simulink model "controllo_giunti_2"  (R2020b)
settings: Solver=FixedStepAuto  StartTime=0.0  StopTime=1  FixedStep=0.001  RelTol=1e-3
libraries: robotcorelib x1
(part 2 of 2)

== matlab function controllo_giunti_2/Subsystem/dq3_dq4 ==
  data: Q input; dQ input; dq3 output; parametri input; dq4 output
function [dq3,dq4] = dq3_dq4(Q,dQ,parametri)
xc1=Q(1);
xc5=Q(2);
q2=Q(3);
dxc1=dQ(1);
dxc5=dQ(2);
dq2=dQ(3);
l=parametri(1);

dq3 =...
(2*dxc5*((2*l + (4*sin(q2)*l^3 - 4*sin(2*q2)*l^2*xc1 - 4*cos(2*q2)*l^2*xc5 - 4*sin(q2)*l*xc1^2 + 8*cos(q2)*l*xc1*xc5 - 12*sin(q2)*l*xc5^2 + 4*xc1^2*xc5 + 4*xc5^3)/(2*(3*l^4 + 4*cos(q2)*l^3*xc1 - 4*sin(q2)*l^3*xc5 - 2*cos(2*q2)*l^2*xc1^2 + 4*sin(2*q2)*l^2*xc1*xc5 + 2*cos(2*q2)*l^2*xc5^2 - 4*cos(q2)*l*xc1^3 + 4*sin(q2)*l*xc1^2*xc5 - 4*cos(q2)*l*xc1*xc5^2 + 4*sin(q2)*l*xc5^3 - xc1^4 - 2*xc1^2*xc5^2 - xc5^4)^(1/2)))/(l^2 - 2*l*xc1 + xc1^2 + xc5^2 - 2*l^2*cos(q2) + 2*l*xc1*cos(q2) - 2*l*xc5*sin(q2)) + ((2*xc5 - 2*l*sin(q2))*(2*l^2*sin(q2) + (3*l^4 + 4*cos(q2)*l^3*xc1 - 4*sin(q2)*l^3*xc5 - 2*cos(2*q2)*l^2*xc1^2 + 4*sin(2*q2)*l^2*xc1*xc5 + 2*cos(2*q2)*l^2*xc5^2 - 4*cos(q2)*l*xc1^3 + 4*sin(q2)*l*xc1^2*xc5 - 4*cos(q2)*l*xc1*xc5^2 + 4*sin(q2)*l*xc5^3 - xc1^4 - 2*xc1^2*xc5^2 - xc5^4)^(1/2) - 2*l*xc5))/(l^2 - 2*l*xc1 + xc1^2 + xc5^2 - 2*l^2*cos(q2) + 2*l*xc1*cos(q2) - 2*l*xc5*sin(q2))^2))/((2*l^2*sin(q2) + (3*l^4 + 4*cos(q2)*l^3*xc1 - 4*sin(q2)*l^3*xc5 - 2*cos(2*q2)*l^2*xc1^2 + 4*sin(2*q2)*l^2*xc1*xc5 + 2*cos(2*q2)*l^2*xc5^2 - 4*cos(q2)*l*xc1^3 + 4*sin(q2)*l*xc1^2*xc5 - 4*cos(q2)*l*xc1*xc5^2 + 4*sin(q2)*l*xc5^3 - xc1^4 - 2*xc1^2*xc5^2 - xc5^4)^(1/2) - 2*l*xc5)^2/(l^2 - 2*l*xc1 + xc1^2 + xc5^2 - 2*l^2*cos(q2) + 2*l*xc1*cos(q2) - 2*l*xc5*sin(q2))^2 + 1) - dq2*((2*(((- 4*sin(q2)*l^3*xc1 - 4*cos(q2)*l^3*xc5 + 4*sin(2*q2)*l^2*xc1^2 + 8*cos(2*q2)*l^2*xc1*xc5 - 4*sin(2*q2)*l^2*xc5^2 + 4*sin(q2)*l*xc1^3 + 4*cos(q2)*l*xc1^2*xc5 + 4*sin(q2)*l*xc1*xc5^2 + 4*cos(q2)*l*xc5^3)/(2*(3*l^4 + 4*cos(q2)*l^3*xc1 - 4*sin(q2)*l^3*xc5 - 2*cos(2*q2)*l^2*xc1^2 + 4*sin(2*q2)*l^2*xc1*xc5 + 2*cos(2*q2)*l^2*xc5^2 - 4*cos(q2)*l*xc1^3 + 4*sin(q2)*l*xc1^2*xc5 - 4*cos(q2)*l*xc1*xc5^2 + 4*sin(q2)*l*xc5^3 - xc1^4 - 2*xc1^2*xc5^2 - xc5^4)^(1/2)) + 2*l^2*cos(q2))/(l^2 - 2*l*xc1 + xc1^2 + xc5^2 - 2*l^2*cos(q2) + 2*l*xc1*cos(q2) - 2*l*xc5*sin(q2)) + ((2*l*xc5*cos(q2) - 2*l^2*sin(q2) + 2*l*xc1*sin(q2))*(2*l^2*sin(q2) + (3*l^4 + 4*cos(q2)*l^3*xc1 - 4*sin(q2)*l^3*xc5 - 2*cos(2*q2)*l^2*xc1^2 + 4*sin(2*q2)*l^2*xc1*xc5 + 2*cos(2*q2)*l^2*xc5^2 - 4*cos(q2)*l*xc1^3 + 4*sin(q2)*l*xc1^2*xc5 - 4*cos(q2)*l*xc1*xc5^2 + 4*sin(q2)*l*xc5^3 - xc1^4 - 2*xc1^2*xc5^2 - xc5^4)^(1/2) - 2*l*xc5))/(l^2 - 2*l*xc1 + xc1^2 + xc5^2 - 2*l^2*cos(q2) + 2*l*xc1*cos(q2) - 2*l*xc5*sin(q2))^2))/((2*l^2*sin(q2) + (3*l^4 + 4*cos(q2)*l^3*xc1 - 4*sin(q2)*l^3*xc5 - 2*cos(2*q2)*l^2*xc1^2 + 4*sin(2*q2)*l^2*xc1*xc5 + 2*cos(2*q2)*l^2*xc5^2 - 4*cos(q2)*l*xc1^3 + 4*sin(q2)*l*xc1^2*xc5 - 4*cos(q2)*l*xc1*xc5^2 + 4*sin(q2)*l*xc5^3 - xc1^4 - 2*xc1^2*xc5^2 - xc5^4)^(1/2) - 2*l*xc5)^2/(l^2 - 2*l*xc1 + xc1^2 + xc5^2 - 2*l^2*cos(q2) + 2*l*xc1*cos(q2) - 2*l*xc5*sin(q2))^2 + 1) + 1) + (2*dxc1*(((2*xc1 - 2*l + 2*l*cos(q2))*(2*l^2*sin(q2) + (3*l^4 + 4*cos(q2)*l^3*xc1 - 4*sin(q2)*l^3*xc5 - 2*cos(2*q2)*l^2*xc1^2 + 4*sin(2*q2)*l^2*xc1*xc5 + 2*cos(2*q2)*l^2*xc5^2 - 4*cos(q2)*l*xc1^3 + 4*sin(q2)*l*xc1^2*xc5 - 4*cos(q2)*l*xc1*xc5^2 + 4*sin(q2)*l*xc5^3 - xc1^4 - 2*xc1^2*xc5^2 - xc5^4)^(1/2) - 2*l*xc5))/(l^2 - 2*l*xc1 + xc1^2 + xc5^2 - 2*l^2*cos(q2) + 2*l*xc1*cos(q2) - 2*l*xc5*sin(q2))^2 + (- 4*cos(q2)*l^3 + 4*cos(2*q2)*l^2*xc1 - 4*sin(2*q2)*l^2*xc5 + 12*cos(q2)*l*xc1^2 - 8*sin(q2)*l*xc1*xc5 + 4*cos(q2)*l*xc5^2 + 4*xc1^3 + 4*xc1*xc5^2)/(2*(l^2 - 2*l*xc1 + xc1^2 + xc5^2 - 2*l^2*cos(q2) + 2*l*xc1*cos(q2) - 2*l*xc5*sin(q2))*(3*l^4 + 4*cos(q2)*l^3*xc1 - 4*sin(q2)*l^3*xc5 - 2*cos(2*q2)*l^2*xc1^2 + 4*sin(2*q2)*l^2*xc1*xc5 + 2*cos(2*q2)*l^2*xc5^2 - 4*cos(q2)*l*xc1^3 + 4*sin(q2)*l*xc1^2*xc5 - 4*cos(q2)*l*xc1*xc5^2 + 4*sin(q2)*l*xc5^3 - xc1^4 - 2*xc1^2*xc5^2 - xc5^4)^(1/2))))/((2*l^2*sin(q2) + (3*l^4 + 4*cos(q2)*l^3*xc1 - 4*sin(q2)*l^3*xc5 - 2*cos(2*q2)*l^2*xc1^2 + 4*sin(2*q2)*l^2*xc1*xc5 + 2*cos(2*q2)*l^2*xc5^2 - 4*cos(q2)*l*xc1^3 + 4*sin(q2)*l*xc1^2*xc5 - 4*cos(q2)*l*xc1*xc5^2 + 4*sin(q2)*l*xc5^3 - xc1^4 - 2*xc1^2*xc5^2 - xc5^4)^(1/2) - 2*l*xc5)^2/(l^2 - 2*l*xc1 + xc1^2 + xc5^2 - 2*l^2*cos(q2) + 2*l*xc1*cos(q2) - 2*l*xc5*sin(q2))^2 + 1);

dq4 =...
 - dxc1*((2*(((2*xc1 - 2*l + 2*l*cos(q2))*((3*l^4 + 4*cos(q2)*l^3*xc1 - 4*sin(q2)*l^3*xc5 - 2*cos(2*q2)*l^2*xc1^2 + 4*sin(2*q2)*l^2*xc1*xc5 + 2*cos(2*q2)*l^2*xc5^2 - 4*cos(q2)*l*xc1^3 + 4*sin(q2)*l*xc1^2*xc5 - 4*cos(q2)*l*xc1*xc5^2 + 4*sin(q2)*l*xc5^3 - xc1^4 - 2*xc1^2*xc5^2 - xc5^4)^(1/2) - 2*l^2*sin(q2) + 2*l*xc5))/(l^2 - 2*l*xc1 + xc1^2 + xc5^2 - 2*l^2*cos(q2) + 2*l*xc1*cos(q2) - 2*l*xc5*sin(q2))^2 + (2*(xc1 + l*cos(q2))*(- l^2 + 2*cos(q2)*l*xc1 - 2*sin(q2)*l*xc5 + xc1^2 + xc5^2))/((l^2 - 2*l*xc1 + xc1^2 + xc5^2 - 2*l^2*cos(q2) + 2*l*xc1*cos(q2) - 2*l*xc5*sin(q2))*(3*l^4 + 4*cos(q2)*l^3*xc1 - 4*sin(q2)*l^3*xc5 - 2*cos(2*q2)*l^2*xc1^2 + 4*sin(2*q2)*l^2*xc1*xc5 + 2*cos(2*q2)*l^2*xc5^2 - 4*cos(q2)*l*xc1^3 + 4*sin(q2)*l*xc1^2*xc5 - 4*cos(q2)*l*xc1*xc5^2 + 4*sin(q2)*l*xc5^3 - xc1^4 - 2*xc1^2*xc5^2 - xc5^4)^(1/2))))/(((3*l^4 + 4*cos(q2)*l^3*xc1 - 4*sin(q2)*l^3*xc5 - 2*cos(2*q2)*l^2*xc1^2 + 4*sin(2*q2)*l^2*xc1*xc5 + 2*cos(2*q2)*l^2*xc5^2 - 4*cos(q2)*l*xc1^3 + 4*sin(q2)*l*xc1^2*xc5 - 4*cos(q2)*l*xc1*xc5^2 + 4*sin(q2)*l*xc5^3 - xc1^4 - 2*xc1^2*xc5^2 - xc5^4)^(1/2) - 2*l^2*sin(q2) + 2*l*xc5)^2/(l^2 - 2*l*xc1 + xc1^2 + xc5^2 - 2*l^2*cos(q2) + 2*l*xc1*cos(q2) - 2*l*xc5*sin(q2))^2 + 1) + (2*(((2*xc1 - 2*l + 2*l*cos(q2))*(2*l^2*sin(q2) + (3*l^4 + 4*cos(q2)*l^3*xc1 - 4*sin(q2)*l^3*xc5 - 2*cos(2*q2)*l^2*xc1^2 + 4*sin(2*q2)*l^2*xc1*xc5 + 2*cos(2*q2)*l^2*xc5^2 - 4*cos(q2)*l*xc1^3 + 4*sin(q2)*l*xc1^2*xc5 - 4*cos(q2)*l*xc1*xc5^2 + 4*sin(q2)*l*xc5^3 - xc1^4 - 2*xc1^2*xc5^2 - xc5^4)^(1/2) - 2*l*xc5))/(l^2 - 2*l*xc1 + xc1^2 + xc5^2 - 2*l^2*cos(q2) + 2*l*xc1*cos(q2) - 2*l*xc5*sin(q2))^2 + (2*(xc1 + l*cos(q2))*(- l^2 + 2*cos(q2)*l*xc1 - 2*sin(q2)*l*xc5 + xc1^2 + xc5^2))/((l^2 - 2*l*xc1 + xc1^2 + xc5^2 - 2*l^2*cos(q2) + 2*l*xc1*cos(q2) - 2*l*xc5*sin(q2))*(3*l^4 + 4*cos(q2)*l^3*xc1 - 4*sin(q2)*l^3*xc5 - 2*cos(2*q2)*l^2*xc1^2 + 4*sin(2*q2)*l^2*xc1*xc5 + 2*cos(2*q2)*l^2*xc5^2 - 4*cos(q2)*l*xc1^3 + 4*sin(q2)*l*xc1^2*xc5 - 4*cos(q2)*l*xc1*xc5^2 + 4*sin(q2)*l*xc5^3 - xc1^4 - 2*xc1^2*xc5^2 - xc5^4)^(1/2))))/((2*l^2*sin(q2) + (3*l^4 + 4*cos(q2)*l^3*xc1 - 4*sin(q2)*l^3*xc5 - 2*cos(2*q2)*l^2*xc1^2 + 4*sin(2*q2)*l^2*xc1*xc5 + 2*cos(2*q2)*l^2*xc5^2 - 4*cos(q2)*l*xc1^3 + 4*sin(q2)*l*xc1^2*xc5 - 4*cos(q2)*l*xc1*xc5^2 + 4*sin(q2)*l*xc5^3 - xc1^4 - 2*xc1^2*xc5^2 - xc5^4)^(1/2) - 2*l*xc5)^2/(l^2 - 2*l*xc1 + xc1^2 + xc5^2 - 2*l^2*cos(q2) + 2*l*xc1*cos(q2) - 2*l*xc5*sin(q2))^2 + 1)) - dxc5*((2*((2*l + (2*sin(q2)*l^3 - 2*sin(2*q2)*l^2*xc1 - 2*cos(2*q2)*l^2*xc5 - 2*sin(q2)*l*xc1^2 + 4*cos(q2)*l*xc1*xc5 - 6*sin(q2)*l*xc5^2 + 2*xc1^2*xc5 + 2*xc5^3)/(3*l^4 + 4*cos(q2)*l^3*xc1 - 4*sin(q2)*l^3*xc5 - 2*cos(2*q2)*l^2*xc1^2 + 4*sin(2*q2)*l^2*xc1*xc5 + 2*cos(2*q2)*l^2*xc5^2 - 4*cos(q2)*l*xc1^3 + 4*sin(q2)*l*xc1^2*xc5 - 4*cos(q2)*l*xc1*xc5^2 + 4*sin(q2)*l*xc5^3 - xc1^4 - 2*xc1^2*xc5^2 - xc5^4)^(1/2))/(l^2 - 2*l*xc1 + xc1^2 + xc5^2 - 2*l^2*cos(q2) + 2*l*xc1*cos(q2) - 2*l*xc5*sin(q2)) + ((2*xc5 - 2*l*sin(q2))*(2*l^2*sin(q2) + (3*l^4 + 4*cos(q2)*l^3*xc1 - 4*sin(q2)*l^3*xc5 - 2*cos(2*q2)*l^2*xc1^2 + 4*sin(2*q2)*l^2*xc1*xc5 + 2*cos(2*q2)*l^2*xc5^2 - 4*cos(q2)*l*xc1^3 + 4*sin(q2)*l*xc1^2*xc5 - 4*cos(q2)*l*xc1*xc5^2 + 4*sin(q2)*l*xc5^3 - xc1^4 - 2*xc1^2*xc5^2 - xc5^4)^(1/2) - 2*l*xc5))/(l^2 - 2*l*xc1 + xc1^2 + xc5^2 - 2*l^2*cos(q2) + 2*l*xc1*cos(q2) - 2*l*xc5*sin(q2))^2))/((2*l^2*sin(q2) + (3*l^4 + 4*cos(q2)*l^3*xc1 - 4*sin(q2)*l^3*xc5 - 2*cos(2*q2)*l^2*xc1^2 + 4*sin(2*q2)*l^2*xc1*xc5 + 2*cos(2*q2)*l^2*xc5^2 - 4*cos(q2)*l*xc1^3 + 4*sin(q2)*l*xc1^2*xc5 - 4*cos(q2)*l*xc1*xc5^2 + 4*sin(q2)*l*xc5^3 - xc1^4 - 2*xc1^2*xc5^2 - xc5^4)^(1/2) - 2*l*xc5)^2/(l^2 - 2*l*xc1 + xc1^2 + xc5^2 - 2*l^2*cos(q2) + 2*l*xc1*cos(q2) - 2*l*xc5*sin(q2))^2 + 1) - (2*((2*l - (2*sin(q2)*l^3 - 2*sin(2*q2)*l^2*xc1 - 2*cos(2*q2)*l^2*xc5 - 2*sin(q2)*l*xc1^2 + 4*cos(q2)*l*xc1*xc5 - 6*sin(q2)*l*xc5^2 + 2*xc1^2*xc5 + 2*xc5^3)/(3*l^4 + 4*cos(q2)*l^3*xc1 - 4*sin(q2)*l^3*xc5 - 2*cos(2*q2)*l^2*xc1^2 + 4*sin(2*q2)*l^2*xc1*xc5 + 2*cos(2*q2)*l^2*xc5^2 - 4*cos(q2)*l*xc1^3 + 4*sin(q2)*l*xc1^2*xc5 - 4*cos(q2)*l*xc1*xc5^2 + 4*sin(q2)*l*xc5^3 - xc1^4 - 2*xc1^2*xc5^2 - xc5^4)^(1/2))/(l^2 - 2*l*xc1 + xc1^2 + xc5^2 - 2*l^2*cos(q2) + 2*l*xc1*cos(q2) - 2*l*xc5*sin(q2)) - ((2*xc5 - 2*l*sin(q2))*((3*l^4 + 4*cos(q2)*l^3*xc1 - 4*sin(q2)*l^3*xc5 - 2*cos(2*q2)*l^2*xc1^2 + 4*sin(2*q2)*l^2*xc1*xc5 + 2*cos(2*q2)*l^2*xc5^2 - 4*cos(q2)*l*xc1^3 + 4*sin(q2)*l*xc1^2*xc5 - 4*cos(q2)*l*xc1*xc5^2 + 4*sin(q2)*l*xc5^3 - xc1^4 - 2*xc1^2*xc5^2 - xc5^4)^(1/2) - 2*l^2*sin(q2) + 2*l*xc5))/(l^2 - 2*l*xc1 + xc1^2 + xc5^2 - 2*l^2*cos(q2) + 2*l*xc1*cos(q2) - 2*l*xc5*sin(q2))^2))/(((3*l^4 + 4*cos(q2)*l^3*xc1 - 4*sin(q2)*l^3*xc5 - 2*cos(2*q2)*l^2*xc1^2 + 4*sin(2*q2)*l^2*xc1*xc5 + 2*cos(2*q2)*l^2*xc5^2 - 4*cos(q2)*l*xc1^3 + 4*sin(q2)*l*xc1^2*xc5 - 4*cos(q2)*l*xc1*xc5^2 + 4*sin(q2)*l*xc5^3 - xc1^4 - 2*xc1^2*xc5^2 - xc5^4)^(1/2) - 2*l^2*sin(q2) + 2*l*xc5)^2/(l^2 - 2*l*xc1 + xc1^2 + xc5^2 - 2*l^2*cos(q2) + 2*l*xc1*cos(q2) - 2*l*xc5*sin(q2))^2 + 1)) - dq2*((2*((2*l^2*cos(q2) - (2*l*(- sin(q2)*l^2*xc1 - cos(q2)*l^2*xc5 + sin(2*q2)*l*xc1^2 + 2*cos(2*q2)*l*xc1*xc5 - sin(2*q2)*l*xc5^2 + sin(q2)*xc1^3 + cos(q2)*xc1^2*xc5 + sin(q2)*xc1*xc5^2 + cos(q2)*xc5^3))/(3*l^4 + 4*cos(q2)*l^3*xc1 - 4*sin(q2)*l^3*xc5 - 2*cos(2*q2)*l^2*xc1^2 + 4*sin(2*q2)*l^2*xc1*xc5 + 2*cos(2*q2)*l^2*xc5^2 - 4*cos(q2)*l*xc1^3 + 4*sin(q2)*l*xc1^2*xc5 - 4*cos(q2)*l*xc1*xc5^2 + 4*sin(q2)*l*xc5^3 - xc1^4 - 2*xc1^2*xc5^2 - xc5^4)^(1/2))/(l^2 - 2*l*xc1 + xc1^2 + xc5^2 - 2*l^2*cos(q2) + 2*l*xc1*cos(q2) - 2*l*xc5*sin(q2)) - (2*l*(xc5*cos(q2) - l*sin(q2) + xc1*sin(q2))*((3*l^4 + 4*cos(q2)*l^3*xc1 - 4*sin(q2)*l^3*xc5 - 2*cos(2*q2)*l^2*xc1^2 + 4*sin(2*q2)*l^2*xc1*xc5 + 2*cos(2*q2)*l^2*xc5^2 - 4*cos(q2)*l*xc1^3 + 4*sin(q2)*l*xc1^2*xc5 - 4*cos(q2)*l*xc1*xc5^2 + 4*sin(q2)*l*xc5^3 - xc1^4 - 2*xc1^2*xc5^2 - xc5^4)^(1/2) - 2*l^2*sin(q2) + 2*l*xc5))/(l^2 - 2*l*xc1 + xc1^2 + xc5^2 - 2*l^2*cos(q2) + 2*l*xc1*cos(q2) - 2*l*xc5*sin(q2))^2))/(((3*l^4 + 4*cos(q2)*l^3*xc1 - 4*sin(q2)*l^3*xc5 - 2*cos(2*q2)*l^2*xc1^2 + 4*sin(2*q2)*l^2*xc1*xc5 + 2*cos(2*q2)*l^2*xc5^2 - 4*cos(q2)*l*xc1^3 + 4*sin(q2)*l*xc1^2*xc5 - 4*cos(q2)*l*xc1*xc5^2 + 4*sin(q2)*l*xc5^3 - xc1^4 - 2*xc1^2*xc5^2 - xc5^4)^(1/2) - 2*l^2*sin(q2) + 2*l*xc5)^2/(l^2 - 2*l*xc1 + xc1^2 + xc5^2 - 2*l^2*cos(q2) + 2*l*xc1*cos(q2) - 2*l*xc5*sin(q2))^2 + 1) - (2*((2*l^2*cos(q2) + (2*l*(- sin(q2)*l^2*xc1 - cos(q2)*l^2*xc5 + sin(2*q2)*l*xc1^2 + 2*cos(2*q2)*l*xc1*xc5 - sin(2*q2)*l*xc5^2 + sin(q2)*xc1^3 + cos(q2)*xc1^2*xc5 + sin(q2)*xc1*xc5^2 + cos(q2)*xc5^3))/(3*l^4 + 4*cos(q2)*l^3*xc1 - 4*sin(q2)*l^3*xc5 - 2*cos(2*q2)*l^2*xc1^2 + 4*sin(2*q2)*l^2*xc1*xc5 + 2*cos(2*q2)*l^2*xc5^2 - 4*cos(q2)*l*xc1^3 + 4*sin(q2)*l*xc1^2*xc5 - 4*cos(q2)*l*xc1*xc5^2 + 4*sin(q2)*l*xc5^3 - xc1^4 - 2*xc1^2*xc5^2 - xc5^4)^(1/2))/(l^2 - 2*l*xc1 + xc1^2 + xc5^2 - 2*l^2*cos(q2) + 2*l*xc1*cos(q2) - 2*l*xc5*sin(q2)) + (2*l*(xc5*cos(q2) - l*sin(q2) + xc1*sin(q2))*(2*l^2*sin(q2) + (3*l^4 + 4*cos(q2)*l^3*xc1 - 4*sin(q2)*l^3*xc5 - 2*cos(2*q2)*l^2*xc1^2 + 4*sin(2*q2)*l^2*xc1*xc5 + 2*cos(2*q2)*l^2*xc5^2 - 4*cos(q2)*l*xc1^3 + 4*sin(q2)*l*xc1^2*xc5 - 4*cos(q2)*l*xc1*xc5^2 + 4*sin(q2)*l*xc5^3 - xc1^4 - 2*xc1^2*xc5^2 - xc5^4)^(1/2) - 2*l*xc5))/(l^2 - 2*l*xc1 + xc1^2 + xc5^2 - 2*l^2*cos(q2) + 2*l*xc1*cos(q2) - 2*l*xc5*sin(q2))^2))/((2*l^2*sin(q2) + (3*l^4 + 4*cos(q2)*l^3*xc1 - 4*sin(q2)*l^3*xc5 - 2*cos(2*q2)*l^2*xc1^2 + 4*sin(2*q2)*l^2*xc1*xc5 + 2*cos(2*q2)*l^2*xc5^2 - 4*cos(q2)*l*xc1^3 + 4*sin(q2)*l*xc1^2*xc5 - 4*cos(q2)*l*xc1*xc5^2 + 4*sin(q2)*l*xc5^3 - xc1^4 - 2*xc1^2*xc5^2 - xc5^4)^(1/2) - 2*l*xc5)^2/(l^2 - 2*l*xc1 + xc1^2 + xc5^2 - 2*l^2*cos(q2) + 2*l*xc1*cos(q2) - 2*l*xc5*sin(q2))^2 + 1));
end

== matlab function controllo_giunti_2/Subsystem/dq3prev_dq4prev ==
  data: Q input; dQ input; dq3 output; parametri input; dq4 output
function [dq3,dq4] = dq3_dq4(Q,dQ,parametri)
xc1=Q(1);
xc5=Q(2);
q2=Q(3);
dxc1=dQ(1);
dxc5=dQ(2);
dq2=dQ(3);
l=parametri(1);

dq3 =...
(2*dxc5*((2*l + (4*sin(q2)*l^3 - 4*sin(2*q2)*l^2*xc1 - 4*cos(2*q2)*l^2*xc5 - 4*sin(q2)*l*xc1^2 + 8*cos(q2)*l*xc1*xc5 - 12*sin(q2)*l*xc5^2 + 4*xc1^2*xc5 + 4*xc5^3)/(2*(3*l^4 + 4*cos(q2)*l^3*xc1 - 4*sin(q2)*l^3*xc5 - 2*cos(2*q2)*l^2*xc1^2 + 4*sin(2*q2)*l^2*xc1*xc5 + 2*cos(2*q2)*l^2*xc5^2 - 4*cos(q2)*l*xc1^3 + 4*sin(q2)*l*xc1^2*xc5 - 4*cos(q2)*l*xc1*xc5^2 + 4*sin(q2)*l*xc5^3 - xc1^4 - 2*xc1^2*xc5^2 - xc5^4)^(1/2)))/(l^2 - 2*l*xc1 + xc1^2 + xc5^2 - 2*l^2*cos(q2) + 2*l*xc1*cos(q2) - 2*l*xc5*sin(q2)) + ((2*xc5 - 2*l*sin(q2))*(2*l^2*sin(q2) + (3*l^4 + 4*cos(q2)*l^3*xc1 - 4*sin(q2)*l^3*xc5 - 2*cos(2*q2)*l^2*xc1^2 + 4*sin(2*q2)*l^2*xc1*xc5 + 2*cos(2*q2)*l^2*xc5^2 - 4*cos(q2)*l*xc1^3 + 4*sin(q2)*l*xc1^2*xc5 - 4*cos(q2)*l*xc1*xc5^2 + 4*sin(q2)*l*xc5^3 - xc1^4 - 2*xc1^2*xc5^2 - xc5^4)^(1/2) - 2*l*xc5))/(l^2 - 2*l*xc1 + xc1^2 + xc5^2 - 2*l^2*cos(q2) + 2*l*xc1*cos(q2) - 2*l*xc5*sin(q2))^2))/((2*l^2*sin(q2) + (3*l^4 + 4*cos(q2)*l^3*xc1 - 4*sin(q2)*l^3*xc5 - 2*cos(2*q2)*l^2*xc1^2 + 4*sin(2*q2)*l^2*xc1*xc5 + 2*cos(2*q2)*l^2*xc5^2 - 4*cos(q2)*l*xc1^3 + 4*sin(q2)*l*xc1^2*xc5 - 4*cos(q2)*l*xc1*xc5^2 + 4*sin(q2)*l*xc5^3 - xc1^4 - 2*xc1^2*xc5^2 - xc5^4)^(1/2) - 2*l*xc5)^2/(l^2 - 2*l*xc1 + xc1^2 + xc5^2 - 2*l^2*cos(q2) + 2*l*xc1*cos(q2) - 2*l*xc5*sin(q2))^2 + 1) - dq2*((2*(((- 4*sin(q2)*l^3*xc1 - 4*cos(q2)*l^3*xc5 + 4*sin(2*q2)*l^2*xc1^2 + 8*cos(2*q2)*l^2*xc1*xc5 - 4*sin(2*q2)*l^2*xc5^2 + 4*sin(q2)*l*xc1^3 + 4*cos(q2)*l*xc1^2*xc5 + 4*sin(q2)*l*xc1*xc5^2 + 4*cos(q2)*l*xc5^3)/(2*(3*l^4 + 4*cos(q2)*l^3*xc1 - 4*sin(q2)*l^3*xc5 - 2*cos(2*q2)*l^2*xc1^2 + 4*sin(2*q2)*l^2*xc1*xc5 + 2*cos(2*q2)*l^2*xc5^2 - 4*cos(q2)*l*xc1^3 + 4*sin(q2)*l*xc1^2*xc5 - 4*cos(q2)*l*xc1*xc5^2 + 4*sin(q2)*l*xc5^3 - xc1^4 - 2*xc1^2*xc5^2 - xc5^4)^(1/2)) + 2*l^2*cos(q2))/(l^2 - 2*l*xc1 + xc1^2 + xc5^2 - 2*l^2*cos(q2) + 2*l*xc1*cos(q2) - 2*l*xc5*sin(q2)) + ((2*l*xc5*cos(q2) - 2*l^2*sin(q2) + 2*l*xc1*sin(q2))*(2*l^2*sin(q2) + (3*l^4 + 4*cos(q2)*l^3*xc1 - 4*sin(q2)*l^3*xc5 - 2*cos(2*q2)*l^2*xc1^2 + 4*sin(2*q2)*l^2*xc1*xc5 + 2*cos(2*q2)*l^2*xc5^2 - 4*cos(q2)*l*xc1^3 + 4*sin(q2)*l*xc1^2*xc5 - 4*cos(q2)*l*xc1*xc5^2 + 4*sin(q2)*l*xc5^3 - xc1^4 - 2*xc1^2*xc5^2 - xc5^4)^(1/2) - 2*l*xc5))/(l^2 - 2*l*xc1 + xc1^2 + xc5^2 - 2*l^2*cos(q2) + 2*l*xc1*cos(q2) - 2*l*xc5*sin(q2))^2))/((2*l^2*sin(q2) + (3*l^4 + 4*cos(q2)*l^3*xc1 - 4*sin(q2)*l^3*xc5 - 2*cos(2*q2)*l^2*xc1^2 + 4*sin(2*q2)*l^2*xc1*xc5 + 2*cos(2*q2)*l^2*xc5^2 - 4*cos(q2)*l*xc1^3 + 4*sin(q2)*l*xc1^2*xc5 - 4*cos(q2)*l*xc1*xc5^2 + 4*sin(q2)*l*xc5^3 - xc1^4 - 2*xc1^2*xc5^2 - xc5^4)^(1/2) - 2*l*xc5)^2/(l^2 - 2*l*xc1 + xc1^2 + xc5^2 - 2*l^2*cos(q2) + 2*l*xc1*cos(q2) - 2*l*xc5*sin(q2))^2 + 1) + 1) + (2*dxc1*(((2*xc1 - 2*l + 2*l*cos(q2))*(2*l^2*sin(q2) + (3*l^4 + 4*cos(q2)*l^3*xc1 - 4*sin(q2)*l^3*xc5 - 2*cos(2*q2)*l^2*xc1^2 + 4*sin(2*q2)*l^2*xc1*xc5 + 2*cos(2*q2)*l^2*xc5^2 - 4*cos(q2)*l*xc1^3 + 4*sin(q2)*l*xc1^2*xc5 - 4*cos(q2)*l*xc1*xc5^2 + 4*sin(q2)*l*xc5^3 - xc1^4 - 2*xc1^2*xc5^2 - xc5^4)^(1/2) - 2*l*xc5))/(l^2 - 2*l*xc1 + xc1^2 + xc5^2 - 2*l^2*cos(q2) + 2*l*xc1*cos(q2) - 2*l*xc5*sin(q2))^2 + (- 4*cos(q2)*l^3 + 4*cos(2*q2)*l^2*xc1 - 4*sin(2*q2)*l^2*xc5 + 12*cos(q2)*l*xc1^2 - 8*sin(q2)*l*xc1*xc5 + 4*cos(q2)*l*xc5^2 + 4*xc1^3 + 4*xc1*xc5^2)/(2*(l^2 - 2*l*xc1 + xc1^2 + xc5^2 - 2*l^2*cos(q2) + 2*l*xc1*cos(q2) - 2*l*xc5*sin(q2))*(3*l^4 + 4*cos(q2)*l^3*xc1 - 4*sin(q2)*l^3*xc5 - 2*cos(2*q2)*l^2*xc1^2 + 4*sin(2*q2)*l^2*xc1*xc5 + 2*cos(2*q2)*l^2*xc5^2 - 4*cos(q2)*l*xc1^3 + 4*sin(q2)*l*xc1^2*xc5 - 4*cos(q2)*l*xc1*xc5^2 + 4*sin(q2)*l*xc5^3 - xc1^4 - 2*xc1^2*xc5^2 - xc5^4)^(1/2))))/((2*l^2*sin(q2) + (3*l^4 + 4*cos(q2)*l^3*xc1 - 4*sin(q2)*l^3*xc5 - 2*cos(2*q2)*l^2*xc1^2 + 4*sin(2*q2)*l^2*xc1*xc5 + 2*cos(2*q2)*l^2*xc5^2 - 4*cos(q2)*l*xc1^3 + 4*sin(q2)*l*xc1^2*xc5 - 4*cos(q2)*l*xc1*xc5^2 + 4*sin(q2)*l*xc5^3 - xc1^4 - 2*xc1^2*xc5^2 - xc5^4)^(1/2) - 2*l*xc5)^2/(l^2 - 2*l*xc1 + xc1^2 + xc5^2 - 2*l^2*cos(q2) + 2*l*xc1*cos(q2) - 2*l*xc5*sin(q2))^2 + 1);

dq4 =...
 - dxc1*((2*(((2*xc1 - 2*l + 2*l*cos(q2))*((3*l^4 + 4*cos(q2)*l^3*xc1 - 4*sin(q2)*l^3*xc5 - 2*cos(2*q2)*l^2*xc1^2 + 4*sin(2*q2)*l^2*xc1*xc5 + 2*cos(2*q2)*l^2*xc5^2 - 4*cos(q2)*l*xc1^3 + 4*sin(q2)*l*xc1^2*xc5 - 4*cos(q2)*l*xc1*xc5^2 + 4*sin(q2)*l*xc5^3 - xc1^4 - 2*xc1^2*xc5^2 - xc5^4)^(1/2) - 2*l^2*sin(q2) + 2*l*xc5))/(l^2 - 2*l*xc1 + xc1^2 + xc5^2 - 2*l^2*cos(q2) + 2*l*xc1*cos(q2) - 2*l*xc5*sin(q2))^2 + (2*(xc1 + l*cos(q2))*(- l^2 + 2*cos(q2)*l*xc1 - 2*sin(q2)*l*xc5 + xc1^2 + xc5^2))/((l^2 - 2*l*xc1 + xc1^2 + xc5^2 - 2*l^2*cos(q2) + 2*l*xc1*cos(q2) - 2*l*xc5*sin(q2))*(3*l^4 + 4*cos(q2)*l^3*xc1 - 4*sin(q2)*l^3*xc5 - 2*cos(2*q2)*l^2*xc1^2 + 4*sin(2*q2)*l^2*xc1*xc5 + 2*cos(2*q2)*l^2*xc5^2 - 4*cos(q2)*l*xc1^3 + 4*sin(q2)*l*xc1^2*xc5 - 4*cos(q2)*l*xc1*xc5^2 + 4*sin(q2)*l*xc5^3 - xc1^4 - 2*xc1^2*xc5^2 - xc5^4)^(1/2))))/(((3*l^4 + 4*cos(q2)*l^3*xc1 - 4*sin(q2)*l^3*xc5 - 2*cos(2*q2)*l^2*xc1^2 + 4*sin(2*q2)*l^2*xc1*xc5 + 2*cos(2*q2)*l^2*xc5^2 - 4*cos(q2)*l*xc1^3 + 4*sin(q2)*l*xc1^2*xc5 - 4*cos(q2)*l*xc1*xc5^2 + 4*sin(q2)*l*xc5^3 - xc1^4 - 2*xc1^2*xc5^2 - xc5^4)^(1/2) - 2*l^2*sin(q2) + 2*l*xc5)^2/(l^2 - 2*l*xc1 + xc1^2 + xc5^2 - 2*l^2*cos(q2) + 2*l*xc1*cos(q2) - 2*l*xc5*sin(q2))^2 + 1) + (2*(((2*xc1 - 2*l + 2*l*cos(q2))*(2*l^2*sin(q2) + (3*l^4 + 4*cos(q2)*l^3*xc1 - 4*sin(q2)*l^3*xc5 - 2*cos(2*q2)*l^2*xc1^2 + 4*sin(2*q2)*l^2*xc1*xc5 + 2*cos(2*q2)*l^2*xc5^2 - 4*cos(q2)*l*xc1^3 + 4*sin(q2)*l*xc1^2*xc5 - 4*cos(q2)*l*xc1*xc5^2 + 4*sin(q2)*l*xc5^3 - xc1^4 - 2*xc1^2*xc5^2 - xc5^4)^(1/2) - 2*l*xc5))/(l^2 - 2*l*xc1 + xc1^2 + xc5^2 - 2*l^2*cos(q2) + 2*l*xc1*cos(q2) - 2*l*xc5*sin(q2))^2 + (2*(xc1 + l*cos(q2))*(- l^2 + 2*cos(q2)*l*xc1 - 2*sin(q2)*l*xc5 + xc1^2 + xc5^2))/((l^2 - 2*l*xc1 + xc1^2 + xc5^2 - 2*l^2*cos(q2) + 2*l*xc1*cos(q2) - 2*l*xc5*sin(q2))*(3*l^4 + 4*cos(q2)*l^3*xc1 - 4*sin(q2)*l^3*xc5 - 2*cos(2*q2)*l^2*xc1^2 + 4*sin(2*q2)*l^2*xc1*xc5 + 2*cos(2*q2)*l^2*xc5^2 - 4*cos(q2)*l*xc1^3 + 4*sin(q2)*l*xc1^2*xc5 - 4*cos(q2)*l*xc1*xc5^2 + 4*sin(q2)*l*xc5^3 - xc1^4 - 2*xc1^2*xc5^2 - xc5^4)^(1/2))))/((2*l^2*sin(q2) + (3*l^4 + 4*cos(q2)*l^3*xc1 - 4*sin(q2)*l^3*xc5 - 2*cos(2*q2)*l^2*xc1^2 + 4*sin(2*q2)*l^2*xc1*xc5 + 2*cos(2*q2)*l^2*xc5^2 - 4*cos(q2)*l*xc1^3 + 4*sin(q2)*l*xc1^2*xc5 - 4*cos(q2)*l*xc1*xc5^2 + 4*sin(q2)*l*xc5^3 - xc1^4 - 2*xc1^2*xc5^2 - xc5^4)^(1/2) - 2*l*xc5)^2/(l^2 - 2*l*xc1 + xc1^2 + xc5^2 - 2*l^2*cos(q2) + 2*l*xc1*cos(q2) - 2*l*xc5*sin(q2))^2 + 1)) - dxc5*((2*((2*l + (2*sin(q2)*l^3 - 2*sin(2*q2)*l^2*xc1 - 2*cos(2*q2)*l^2*xc5 - 2*sin(q2)*l*xc1^2 + 4*cos(q2)*l*xc1*xc5 - 6*sin(q2)*l*xc5^2 + 2*xc1^2*xc5 + 2*xc5^3)/(3*l^4 + 4*cos(q2)*l^3*xc1 - 4*sin(q2)*l^3*xc5 - 2*cos(2*q2)*l^2*xc1^2 + 4*sin(2*q2)*l^2*xc1*xc5 + 2*cos(2*q2)*l^2*xc5^2 - 4*cos(q2)*l*xc1^3 + 4*sin(q2)*l*xc1^2*xc5 - 4*cos(q2)*l*xc1*xc5^2 + 4*sin(q2)*l*xc5^3 - xc1^4 - 2*xc1^2*xc5^2 - xc5^4)^(1/2))/(l^2 - 2*l*xc1 + xc1^2 + xc5^2 - 2*l^2*cos(q2) + 2*l*xc1*cos(q2) - 2*l*xc5*sin(q2)) + ((2*xc5 - 2*l*sin(q2))*(2*l^2*sin(q2) + (3*l^4 + 4*cos(q2)*l^3*xc1 - 4*sin(q2)*l^3*xc5 - 2*cos(2*q2)*l^2*xc1^2 + 4*sin(2*q2)*l^2*xc1*xc5 + 2*cos(2*q2)*l^2*xc5^2 - 4*cos(q2)*l*xc1^3 + 4*sin(q2)*l*xc1^2*xc5 - 4*cos(q2)*l*xc1*xc5^2 + 4*sin(q2)*l*xc5^3 - xc1^4 - 2*xc1^2*xc5^2 - xc5^4)^(1/2) - 2*l*xc5))/(l^2 - 2*l*xc1 + xc1^2 + xc5^2 - 2*l^2*cos(q2) + 2*l*xc1*cos(q2) - 2*l*xc5*sin(q2))^2))/((2*l^2*sin(q2) + (3*l^4 + 4*cos(q2)*l^3*xc1 - 4*sin(q2)*l^3*xc5 - 2*cos(2*q2)*l^2*xc1^2 + 4*sin(2*q2)*l^2*xc1*xc5 + 2*cos(2*q2)*l^2*xc5^2 - 4*cos(q2)*l*xc1^3 + 4*sin(q2)*l*xc1^2*xc5 - 4*cos(q2)*l*xc1*xc5^2 + 4*sin(q2)*l*xc5^3 - xc1^4 - 2*xc1^2*xc5^2 - xc5^4)^(1/2) - 2*l*xc5)^2/(l^2 - 2*l*xc1 + xc1^2 + xc5^2 - 2*l^2*cos(q2) + 2*l*xc1*cos(q2) - 2*l*xc5*sin(q2))^2 + 1) - (2*((2*l - (2*sin(q2)*l^3 - 2*sin(2*q2)*l^2*xc1 - 2*cos(2*q2)*l^2*xc5 - 2*sin(q2)*l*xc1^2 + 4*cos(q2)*l*xc1*xc5 - 6*sin(q2)*l*xc5^2 + 2*xc1^2*xc5 + 2*xc5^3)/(3*l^4 + 4*cos(q2)*l^3*xc1 - 4*sin(q2)*l^3*xc5 - 2*cos(2*q2)*l^2*xc1^2 + 4*sin(2*q2)*l^2*xc1*xc5 + 2*cos(2*q2)*l^2*xc5^2 - 4*cos(q2)*l*xc1^3 + 4*sin(q2)*l*xc1^2*xc5 - 4*cos(q2)*l*xc1*xc5^2 + 4*sin(q2)*l*xc5^3 - xc1^4 - 2*xc1^2*xc5^2 - xc5^4)^(1/2))/(l^2 - 2*l*xc1 + xc1^2 + xc5^2 - 2*l^2*cos(q2) + 2*l*xc1*cos(q2) - 2*l*xc5*sin(q2)) - ((2*xc5 - 2*l*sin(q2))*((3*l^4 + 4*cos(q2)*l^3*xc1 - 4*sin(q2)*l^3*xc5 - 2*cos(2*q2)*l^2*xc1^2 + 4*sin(2*q2)*l^2*xc1*xc5 + 2*cos(2*q2)*l^2*xc5^2 - 4*cos(q2)*l*xc1^3 + 4*sin(q2)*l*xc1^2*xc5 - 4*cos(q2)*l*xc1*xc5^2 + 4*sin(q2)*l*xc5^3 - xc1^4 - 2*xc1^2*xc5^2 - xc5^4)^(1/2) - 2*l^2*sin(q2) + 2*l*xc5))/(l^2 - 2*l*xc1 + xc1^2 + xc5^2 - 2*l^2*cos(q2) + 2*l*xc1*cos(q2) - 2*l*xc5*sin(q2))^2))/(((3*l^4 + 4*cos(q2)*l^3*xc1 - 4*sin(q2)*l^3*xc5 - 2*cos(2*q2)*l^2*xc1^2 + 4*sin(2*q2)*l^2*xc1*xc5 + 2*cos(2*q2)*l^2*xc5^2 - 4*cos(q2)*l*xc1^3 + 4*sin(q2)*l*xc1^2*xc5 - 4*cos(q2)*l*xc1*xc5^2 + 4*sin(q2)*l*xc5^3 - xc1^4 - 2*xc1^2*xc5^2 - xc5^4)^(1/2) - 2*l^2*sin(q2) + 2*l*xc5)^2/(l^2 - 2*l*xc1 + xc1^2 + xc5^2 - 2*l^2*cos(q2) + 2*l*xc1*cos(q2) - 2*l*xc5*sin(q2))^2 + 1)) - dq2*((2*((2*l^2*cos(q2) - (2*l*(- sin(q2)*l^2*xc1 - cos(q2)*l^2*xc5 + sin(2*q2)*l*xc1^2 + 2*cos(2*q2)*l*xc1*xc5 - sin(2*q2)*l*xc5^2 + sin(q2)*xc1^3 + cos(q2)*xc1^2*xc5 + sin(q2)*xc1*xc5^2 + cos(q2)*xc5^3))/(3*l^4 + 4*cos(q2)*l^3*xc1 - 4*sin(q2)*l^3*xc5 - 2*cos(2*q2)*l^2*xc1^2 + 4*sin(2*q2)*l^2*xc1*xc5 + 2*cos(2*q2)*l^2*xc5^2 - 4*cos(q2)*l*xc1^3 + 4*sin(q2)*l*xc1^2*xc5 - 4*cos(q2)*l*xc1*xc5^2 + 4*sin(q2)*l*xc5^3 - xc1^4 - 2*xc1^2*xc5^2 - xc5^4)^(1/2))/(l^2 - 2*l*xc1 + xc1^2 + xc5^2 - 2*l^2*cos(q2) + 2*l*xc1*cos(q2) - 2*l*xc5*sin(q2)) - (2*l*(xc5*cos(q2) - l*sin(q2) + xc1*sin(q2))*((3*l^4 + 4*cos(q2)*l^3*xc1 - 4*sin(q2)*l^3*xc5 - 2*cos(2*q2)*l^2*xc1^2 + 4*sin(2*q2)*l^2*xc1*xc5 + 2*cos(2*q2)*l^2*xc5^2 - 4*cos(q2)*l*xc1^3 + 4*sin(q2)*l*xc1^2*xc5 - 4*cos(q2)*l*xc1*xc5^2 + 4*sin(q2)*l*xc5^3 - xc1^4 - 2*xc1^2*xc5^2 - xc5^4)^(1/2) - 2*l^2*sin(q2) + 2*l*xc5))/(l^2 - 2*l*xc1 + xc1^2 + xc5^2 - 2*l^2*cos(q2) + 2*l*xc1*cos(q2) - 2*l*xc5*sin(q2))^2))/(((3*l^4 + 4*cos(q2)*l^3*xc1 - 4*sin(q2)*l^3*xc5 - 2*cos(2*q2)*l^2*xc1^2 + 4*sin(2*q2)*l^2*xc1*xc5 + 2*cos(2*q2)*l^2*xc5^2 - 4*cos(q2)*l*xc1^3 + 4*sin(q2)*l*xc1^2*xc5 - 4*cos(q2)*l*xc1*xc5^2 + 4*sin(q2)*l*xc5^3 - xc1^4 - 2*xc1^2*xc5^2 - xc5^4)^(1/2) - 2*l^2*sin(q2) + 2*l*xc5)^2/(l^2 - 2*l*xc1 + xc1^2 + xc5^2 - 2*l^2*cos(q2) + 2*l*xc1*cos(q2) - 2*l*xc5*sin(q2))^2 + 1) - (2*((2*l^2*cos(q2) + (2*l*(- sin(q2)*l^2*xc1 - cos(q2)*l^2*xc5 + sin(2*q2)*l*xc1^2 + 2*cos(2*q2)*l*xc1*xc5 - sin(2*q2)*l*xc5^2 + sin(q2)*xc1^3 + cos(q2)*xc1^2*xc5 + sin(q2)*xc1*xc5^2 + cos(q2)*xc5^3))/(3*l^4 + 4*cos(q2)*l^3*xc1 - 4*sin(q2)*l^3*xc5 - 2*cos(2*q2)*l^2*xc1^2 + 4*sin(2*q2)*l^2*xc1*xc5 + 2*cos(2*q2)*l^2*xc5^2 - 4*cos(q2)*l*xc1^3 + 4*sin(q2)*l*xc1^2*xc5 - 4*cos(q2)*l*xc1*xc5^2 + 4*sin(q2)*l*xc5^3 - xc1^4 - 2*xc1^2*xc5^2 - xc5^4)^(1/2))/(l^2 - 2*l*xc1 + xc1^2 + xc5^2 - 2*l^2*cos(q2) + 2*l*xc1*cos(q2) - 2*l*xc5*sin(q2)) + (2*l*(xc5*cos(q2) - l*sin(q2) + xc1*sin(q2))*(2*l^2*sin(q2) + (3*l^4 + 4*cos(q2)*l^3*xc1 - 4*sin(q2)*l^3*xc5 - 2*cos(2*q2)*l^2*xc1^2 + 4*sin(2*q2)*l^2*xc1*xc5 + 2*cos(2*q2)*l^2*xc5^2 - 4*cos(q2)*l*xc1^3 + 4*sin(q2)*l*xc1^2*xc5 - 4*cos(q2)*l*xc1*xc5^2 + 4*sin(q2)*l*xc5^3 - xc1^4 - 2*xc1^2*xc5^2 - xc5^4)^(1/2) - 2*l*xc5))/(l^2 - 2*l*xc1 + xc1^2 + xc5^2 - 2*l^2*cos(q2) + 2*l*xc1*cos(q2) - 2*l*xc5*sin(q2))^2))/((2*l^2*sin(q2) + (3*l^4 + 4*cos(q2)*l^3*xc1 - 4*sin(q2)*l^3*xc5 - 2*cos(2*q2)*l^2*xc1^2 + 4*sin(2*q2)*l^2*xc1*xc5 + 2*cos(2*q2)*l^2*xc5^2 - 4*cos(q2)*l*xc1^3 + 4*sin(q2)*l*xc1^2*xc5 - 4*cos(q2)*l*xc1*xc5^2 + 4*sin(q2)*l*xc5^3 - xc1^4 - 2*xc1^2*xc5^2 - xc5^4)^(1/2) - 2*l*xc5)^2/(l^2 - 2*l*xc1 + xc1^2 + xc5^2 - 2*l^2*cos(q2) + 2*l*xc1*cos(q2) - 2*l*xc5*sin(q2))^2 + 1));
end

== matlab function controllo_giunti_2/Subsystem/ddq3_ddq4 ==
  data: dq3 input; ddq3 output; dq4 input; dq3_prev input; dq4_prev input; dt input; ddq4 output
function [ddq3,ddq4] = ddq3_ddq4(dq3,dq4,dq3_prev,dq4_prev,dt)

ddq3=(dq3-dq3_prev)/dt;
ddq4=(dq4-dq4_prev)/dt;
end
